simulink model "suspension7DOF"  (R2025b)
settings: Solver=ode5  StartTime=0.0  StopTime=10.0  FixedStep=0.001  RelTol=1e-3
InitFcn:
  | % 悬架参数
  | ksfl =  20000;
  | ksfr = ksfl;
  | ksrl =  20000;
  | ksrr = ksrl;
  | 
  | csfl = 1100;
  | csfr = 1100;
  | csrl = 1100;
  | csrr = 1100;
undefined symbols (not defined in the file): road
settings Model: Creator=23649  LastModifiedBy=23649

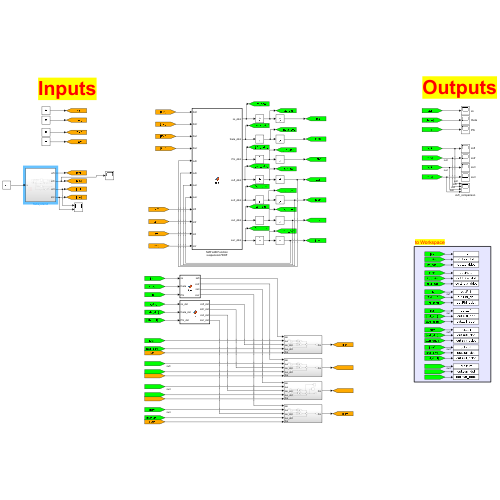
[thumbnail: Simulink's stored preview of the top-level diagram]
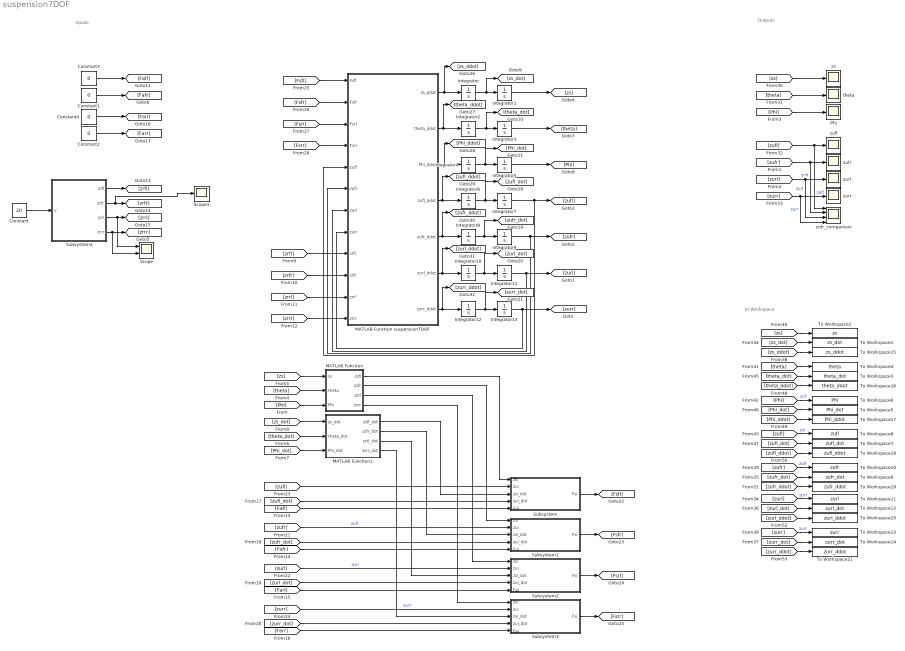
== system suspension7DOF ==
  note: Inputs
  note: Outputs
  note: to Workspace
  Constant : Constant  Value=20
  Constant{1..4} (4 alike) : Constant  Value=0
  Integrator{,1..13} (14 alike) : Integrator
  MATLAB Function : MATLAB Function  TreatAsAtomicUnit=on
  MATLAB Function suspension7DOF : MATLAB Function  TreatAsAtomicUnit=on
  MATLAB Function1 : MATLAB Function  TreatAsAtomicUnit=on
  Phi : Scope
      settings: ActiveDisplayYMinimum=-0.0087264176221422858  ActiveDisplayYMaximum=0.021115769306995449  DataLoggingVariableName=ScopeData7
  Scope : Scope  NumInputPorts=2
      settings: ActiveDisplayYMinimum=-0.0707302288699563  ActiveDisplayYMaximum=0.0028881749124079481  DataLoggingVariableName=ScopeData10
  Scope1 : Scope
      settings: ActiveDisplayYMinimum=-1  ActiveDisplayYMaximum=1  DataLoggingVariableName=ScopeData11
  Subsystem : Subsystem
  Subsystem1 : Subsystem
  Subsystem2 : Subsystem
  Subsystem3 : Subsystem
  Subsystem4 : Subsystem
  To Workspace1 : ToWorkspace  VariableName=zs_dot  SampleTime=-1
  To Workspace10 : ToWorkspace  VariableName=zufr  SampleTime=-1
  To Workspace11 : ToWorkspace  VariableName=zurl  SampleTime=-1
  To Workspace12 : ToWorkspace  VariableName=zurl_dot  SampleTime=-1
  To Workspace13 : ToWorkspace  VariableName=zurr  SampleTime=-1
  To Workspace14 : ToWorkspace  VariableName=zurr_dot  SampleTime=-1
  To Workspace15 : ToWorkspace  VariableName=zs_ddot  SampleTime=-1
  To Workspace16 : ToWorkspace  VariableName=theta_ddot  SampleTime=-1
  To Workspace17 : ToWorkspace  VariableName=Phi_ddot  SampleTime=-1
  To Workspace18 : ToWorkspace  VariableName=zufl_ddot  SampleTime=-1
  To Workspace19 : ToWorkspace  VariableName=zufr_ddot  SampleTime=-1
  To Workspace2 : ToWorkspace  VariableName=zs  SampleTime=-1
  To Workspace20 : ToWorkspace  VariableName=zurl_ddot  SampleTime=-1
  To Workspace21 : ToWorkspace  VariableName=zurr_ddot  SampleTime=-1
  To Workspace3 : ToWorkspace  VariableName=theta_dot  SampleTime=-1
  To Workspace4 : ToWorkspace  VariableName=theta  SampleTime=-1
  To Workspace5 : ToWorkspace  VariableName=Phi_dot  SampleTime=-1
  To Workspace6 : ToWorkspace  VariableName=Phi  SampleTime=-1
  To Workspace7 : ToWorkspace  VariableName=zufl_dot  SampleTime=-1
  To Workspace8 : ToWorkspace  VariableName=zufl  SampleTime=-1
  To Workspace9 : ToWorkspace  VariableName=zufr_dot  SampleTime=-1
  theta : Scope
      settings: ActiveDisplayYMinimum=-0.012479397367141442  ActiveDisplayYMaximum=0.012968504515283082
  zs : Scope
      settings: ActiveDisplayYMinimum=-0.038035702406532847  ActiveDisplayYMaximum=0.14136596040152494  DataLoggingVariableName=ScopeData2
  zufl : Scope
      settings: ActiveDisplayYMinimum=-1.3673893789653644  ActiveDisplayYMaximum=1.3691796129847056
  zufr : Scope
      settings: ActiveDisplayYMinimum=-1.3540132201466146  ActiveDisplayYMaximum=1.3380491130807826  DataLoggingVariableName=ScopeData5
  zufr_comparison : Scope  NumInputPorts=4
      settings: ActiveDisplayYMinimum=-0.078530307125556281  ActiveDisplayYMaximum=0.21658201066899388  DataLoggingVariableName=ScopeData4
  zurl : Scope
      settings: ActiveDisplayYMinimum=-1.3540132201466146  ActiveDisplayYMaximum=1.3380491130807826  DataLoggingVariableName=ScopeData6
  zurr : Scope
      settings: ActiveDisplayYMinimum=-1.3540132201466146  ActiveDisplayYMaximum=1.3380491130807826  DataLoggingVariableName=ScopeData3
  wires:
  Constant3/1 -> [Fafl]
  Constant1/1 -> [Fafr]
  [zs] -> zs/1
  [theta] -> theta/1
  [zufl] -> zufl/1, zufr_comparison/1  "zufl"
  [zurr] -> zufr_comparison/4, zurr/1  "zurr"
  MATLAB Function suspension7DOF/7(zurr_ddot) -> Integrator12/1, [zurr_ddot]
  MATLAB Function suspension7DOF/6(zurl_ddot) -> Integrator10/1, [zurl_ddot]
  MATLAB Function suspension7DOF/5(zufr_ddot) -> [zufr_ddot], Integrator8/1
  MATLAB Function suspension7DOF/4(zufl_ddot) -> Integrator6/1, [zufl_ddot]
  MATLAB Function suspension7DOF/1(zs_ddot) -> [zs_ddot], Integrator/1
  Integrator/1 -> [zs_dot], Integrator1/1
  Integrator2/1 -> [theta_dot], Integrator3/1
  Integrator4/1 -> [Phi_dot], Integrator5/1
  Integrator6/1 -> Integrator7/1, [zufl_dot]
  Integrator8/1 -> [zufr_dot], Integrator9/1
  Integrator10/1 -> [zurl_dot], Integrator11/1
  Integrator12/1 -> [zurr_dot], Integrator13/1
  MATLAB Function suspension7DOF/3(Phi_ddot) -> [Phi_ddot], Integrator4/1
  MATLAB Function suspension7DOF/2(theta_ddot) -> Integrator2/1, [theta_ddot]
  Integrator13/1 -> [zurr], MATLAB Function suspension7DOF/8(zurr)
  Integrator11/1 -> [zurl], MATLAB Function suspension7DOF/7(zurl)
  Integrator9/1 -> [zufr], MATLAB Function suspension7DOF/6(zufr)
  Integrator7/1 -> [zufl], MATLAB Function suspension7DOF/5(zufl)
  [zufr] -> zufr_comparison/2, zufr/1  "zufr"
  [zurl] -> zurl/1, zufr_comparison/3  "zurl"
  [Phi] -> Phi/1
  Integrator5/1 -> [Phi]
  Integrator3/1 -> [theta]
  Integrator1/1 -> [zs]
  [zs] -> MATLAB Function/1(zs)
  [theta] -> MATLAB Function/2(theta)
  [Phi] -> MATLAB Function/3(Phi)
  [zs_dot] -> MATLAB Function1/1(zs_dot)
  [theta_dot] -> MATLAB Function1/2(theta_dot)
  [Phi_dot] -> MATLAB Function1/3(Phi_dot)
  [zrfl] -> MATLAB Function suspension7DOF/9(zrfl)
  [zrfr] -> MATLAB Function suspension7DOF/10(zrfr)
  [zrrl] -> MATLAB Function suspension7DOF/11(zrrl)
  [zrrr] -> MATLAB Function suspension7DOF/12(zrrr)
  MATLAB Function/1(zsfl) -> Subsystem/1(zsi)
  [zufl] -> Subsystem/2(zui)
  [zufl_dot] -> Subsystem/4(zui_dot)
  [Fafl] -> Subsystem/5(Fai)
  Subsystem/1(Fsi) -> [Fsfl]
  Constant2/1 -> [Farr]
  Constant4/1 -> [Farl]
  MATLAB Function/2(zsfr) -> Subsystem1/1(zsi)
  MATLAB Function/3(zsrl) -> Subsystem2/1(zsi)
  MATLAB Function/4(zsrr) -> Subsystem3/1(zsi)
  MATLAB Function1/1(zsfl_dot) -> Subsystem/3(zsi_dot)
  MATLAB Function1/2(zsfr_dot) -> Subsystem1/3(zsi_dot)
  MATLAB Function1/3(zsrl_dot) -> Subsystem2/3(zsi_dot)
  MATLAB Function1/4(zsrr_dot) -> Subsystem3/3(zsi_dot)
  [zufr_dot] -> Subsystem1/4(zui_dot)
  [zurr_dot] -> Subsystem3/4(zui_dot)
  [zurl_dot] -> Subsystem2/4(zui_dot)
  [Farr] -> Subsystem3/5(Fai)
  [Farl] -> Subsystem2/5(Fai)
  [Fafr] -> Subsystem1/5(Fai)
  [zufr] -> Subsystem1/2(zui)  "zufr"
  [zurl] -> Subsystem2/2(zui)  "zurl"
  [zurr] -> Subsystem3/2(zui)  "zurr"
  Subsystem3/1(Fsi) -> [Fsrr]
  Subsystem2/1(Fsi) -> [Fsrl]
  Subsystem1/1(Fsi) -> [Fsfr]
  [Fsfl] -> MATLAB Function suspension7DOF/1(Fsfl)
  [Fsfr] -> MATLAB Function suspension7DOF/2(Fsfr)
  [Fsrl] -> MATLAB Function suspension7DOF/3(Fsrl)
  [Fsrr] -> MATLAB Function suspension7DOF/4(Fsrr)
  Subsystem4/1(zrfl) -> [zrfl]
  Subsystem4/2(zrfr) -> Scope1/1, [zrfr]
  Subsystem4/3(zrrl) -> Scope/1, [zrrl]
  Constant/1 -> Subsystem4/1(v)
  [zufl] -> To Workspace8/1  "zur"
  [zs] -> To Workspace2/1
  [zufl_dot] -> To Workspace7/1
  [Phi] -> To Workspace6/1  "zuf"
  [theta] -> To Workspace4/1
  [Phi_dot] -> To Workspace5/1
  [theta_dot] -> To Workspace3/1
  [zs_dot] -> To Workspace1/1
  [zurr_dot] -> To Workspace14/1
  [zurr] -> To Workspace13/1  "zurr"
  [zurl_dot] -> To Workspace12/1
  [zurl] -> To Workspace11/1  "zurl"
  [zufr_dot] -> To Workspace9/1
  [zufr] -> To Workspace10/1  "zufr"
  [zs_ddot] -> To Workspace15/1
  [theta_ddot] -> To Workspace16/1
  [Phi_ddot] -> To Workspace17/1
  [zufl_ddot] -> To Workspace18/1
  [zufr_ddot] -> To Workspace19/1
  [zurl_ddot] -> To Workspace20/1
  [zurr_ddot] -> To Workspace21/1
  Subsystem4/4(zrrr) -> Scope/2, [zrrr]

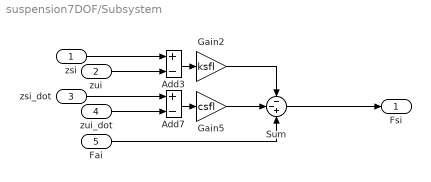
== system suspension7DOF/Subsystem ==
  zsi : Inport
  zui : Inport  Port=2
  zsi_dot : Inport  Port=3
  zui_dot : Inport  Port=4
  Fai : Inport  Port=5
  Add3 : Sum  Inputs=+-
  Add7 : Sum  Inputs=+-
  Gain2 : Gain  Gain=ksfl
  Gain5 : Gain  Gain=csfl
  Sum : Sum  Inputs=--+
  Fsi : Outport
  wires:
  Gain2/1 -> Sum/1
  zsi_dot/1 -> Add7/1
  zsi/1 -> Add3/1
  Add7/1 -> Gain5/1
  zui/1 -> Add3/2
  Add3/1 -> Gain2/1
  Gain5/1 -> Sum/2
  Fai/1 -> Sum/3
  Sum/1 -> Fsi/1
  zui_dot/1 -> Add7/2

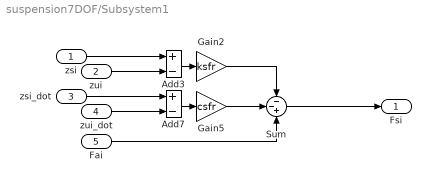
== system suspension7DOF/Subsystem1 ==
  zsi : Inport
  zui : Inport  Port=2
  zsi_dot : Inport  Port=3
  zui_dot : Inport  Port=4
  Fai : Inport  Port=5
  Add3 : Sum  Inputs=+-
  Add7 : Sum  Inputs=+-
  Gain2 : Gain  Gain=ksfr
  Gain5 : Gain  Gain=csfr
  Sum : Sum  Inputs=--+
  Fsi : Outport
  wires:
  zui_dot/1 -> Add7/2
  Sum/1 -> Fsi/1
  Fai/1 -> Sum/3
  Gain5/1 -> Sum/2
  Add3/1 -> Gain2/1
  zui/1 -> Add3/2
  Add7/1 -> Gain5/1
  zsi/1 -> Add3/1
  zsi_dot/1 -> Add7/1
  Gain2/1 -> Sum/1

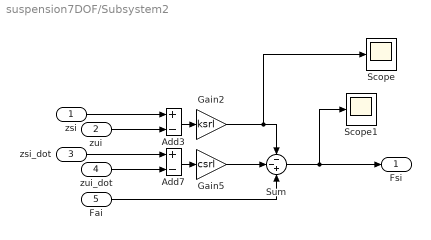
== system suspension7DOF/Subsystem2 ==
  zsi : Inport
  zui : Inport  Port=2
  zsi_dot : Inport  Port=3
  zui_dot : Inport  Port=4
  Fai : Inport  Port=5
  Add3 : Sum  Inputs=+-
  Add7 : Sum  Inputs=+-
  Gain2 : Gain  Gain=ksrl
  Gain5 : Gain  Gain=csrl
  Scope : Scope
      settings: ActiveDisplayYMinimum=-1  ActiveDisplayYMaximum=1  DataLoggingVariableName=ScopeData8
  Scope1 : Scope
      settings: ActiveDisplayYMinimum=-8980.6897654374643  ActiveDisplayYMaximum=18965.2502378485  DataLoggingVariableName=ScopeData9
  Sum : Sum  Inputs=--+
  Fsi : Outport
  wires:
  Gain2/1 -> Scope/1, Sum/1
  zsi_dot/1 -> Add7/1
  zsi/1 -> Add3/1
  Add7/1 -> Gain5/1
  zui/1 -> Add3/2
  Add3/1 -> Gain2/1
  Gain5/1 -> Sum/2
  Fai/1 -> Sum/3
  Sum/1 -> Scope1/1, Fsi/1
  zui_dot/1 -> Add7/2

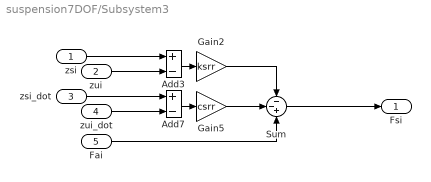
== system suspension7DOF/Subsystem3 ==
  zsi : Inport
  zui : Inport  Port=2
  zsi_dot : Inport  Port=3
  zui_dot : Inport  Port=4
  Fai : Inport  Port=5
  Add3 : Sum  Inputs=+-
  Add7 : Sum  Inputs=+-
  Gain2 : Gain  Gain=ksrr
  Gain5 : Gain  Gain=csrr
  Sum : Sum  Inputs=--+
  Fsi : Outport
  wires:
  zui_dot/1 -> Add7/2
  Sum/1 -> Fsi/1
  Fai/1 -> Sum/3
  Gain5/1 -> Sum/2
  Add3/1 -> Gain2/1
  zui/1 -> Add3/2
  Add7/1 -> Gain5/1
  zsi/1 -> Add3/1
  zsi_dot/1 -> Add7/1
  Gain2/1 -> Sum/1

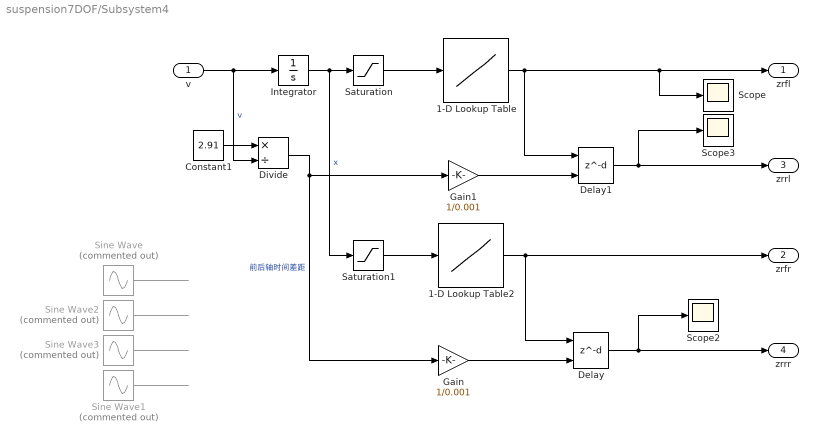
== system suspension7DOF/Subsystem4 ==
  v : Inport
  1-D Lookup Table : Lookup_n-D  NumberOfTableDimensions=1  BreakpointsForDimension1=road.x  Table=road.z_L  ExtrapMethod=Clip  InternalRulePriority=Speed  RndMeth=Simplest
  1-D Lookup Table2 : Lookup_n-D  NumberOfTableDimensions=1  BreakpointsForDimension1=road.x  Table=road.z_R  ExtrapMethod=Clip  InternalRulePriority=Speed  RndMeth=Simplest
  Constant1 : Constant  Value=2.91
  Delay : Delay  DelayLengthSource=Input port  DelayLength=1  DelayLengthUpperLimit=1000  InputProcessing=Columns as channels (frame based)
      settings: InputPortMap=u0,p1
  Delay1 : Delay  DelayLengthSource=Input port  DelayLength=1  DelayLengthUpperLimit=1000  InputProcessing=Columns as channels (frame based)
      settings: InputPortMap=u0,p1
  Divide : Product  Inputs=*/
  Gain : Gain  Gain=1/0.001
  Gain1 : Gain  Gain=1/0.001
  Integrator : Integrator
  Saturation : Saturate  UpperLimit=road.L-road.dx  LowerLimit=0
  Saturation1 : Saturate  UpperLimit=road.L-road.dx  LowerLimit=0
  Scope : Scope
      settings: ActiveDisplayYMinimum=-1  ActiveDisplayYMaximum=1  DataLoggingVariableName=ScopeData12
  Scope2 : Scope
      settings: ActiveDisplayYMinimum=-1  ActiveDisplayYMaximum=1  DataLoggingVariableName=ScopeData14
  Scope3 : Scope
      settings: ActiveDisplayYMinimum=-0.089220015836879121  ActiveDisplayYMaximum=0.19824348779036427  DataLoggingVariableName=ScopeData15
  Sine Wave : Sin  Commented=on  Frequency=5  SampleTime=0
  Sine Wave1 : Sin  Commented=on  Frequency=5  Phase=7  SampleTime=0
  Sine Wave2 : Sin  Commented=on  Frequency=5  SampleTime=0
  Sine Wave3 : Sin  Commented=on  Frequency=5  Phase=12  SampleTime=0
  zrfl : Outport
  zrfr : Outport  Port=2
  zrrl : Outport  Port=3
  zrrr : Outport  Port=4
  wires:
  v/1 -> Integrator/1, Divide/2  "v"
  Integrator/1 -> Saturation/1, Saturation1/1  "x"
  Saturation/1 -> 1-D Lookup Table/1
  Saturation1/1 -> 1-D Lookup Table2/1
  Sine Wave2/1 -> ?
  Sine Wave1/1 -> ?
  Sine Wave/1 -> ?
  Sine Wave3/1 -> ?
  Delay/1 -> Scope2/1, zrrr/1
  Constant1/1 -> Divide/1
  Divide/1 -> Gain1/1, Gain/1  "前后轴时间差距"
  Gain/1 -> Delay/2
  1-D Lookup Table2/1 -> Delay/1, zrfr/1
  1-D Lookup Table/1 -> Delay1/1, Scope/1, zrfl/1
  Gain1/1 -> Delay1/2
  Delay1/1 -> zrrl/1, Scope3/1

== matlab function suspension7DOF/MATLAB Function ==
  data: zs input; zsfl output; theta input; Phi input; zsfr output; zsrl output; zsrr output
function [zsfl, zsfr, zsrl, zsrr] = fcn(zs, theta, Phi)
    
    lf = 1110*0.001;
    L = 2866*0.001;
    % lr = L-lf;
    lr = lf;
    Bf = 1550*0.001;
    Br = Bf;


    zsfl = zs - lf*theta + Bf/2*Phi;
    zsfr = zs - lf*theta - Bf/2*Phi;
    zsrl = zs + lr*theta + Br/2*Phi;
    zsrr = zs + lr*theta - Br/2*Phi;

end

== matlab function suspension7DOF/MATLAB Function suspension7DOF ==
  data: Fsfl input; zs_ddot output; theta_ddot output; Phi_ddot output; zufl_ddot output; zufr_ddot output; zurl_ddot output; zurr_ddot output; Fsfr input; Fsrl input; Fsrr input; zufl input; zufr input; zurl input; zurr input; zrfl input; zrfr input; zrrl input; zrrr input
function [zs_ddot,theta_ddot,Phi_ddot,zufl_ddot,zufr_ddot,zurl_ddot,zurr_ddot] = fcn(Fsfl,Fsfr,Fsrl,Fsrr,zufl,zufr,zurl,zurr,zrfl,zrfr,zrrl,zrrr)
    % 物理参数
    m_s = 1370;
    Iy = 1972.8;
    Ix = 671.3;
    lf = 1110*0.001;
    L = 2866*0.001;
    lr = L-lf;
    Bf = 1550*0.001;
    Br = Bf;
    m_ufl = 89.9/2;
    m_ufr = m_ufl;
    m_url = 65.2/2;
    m_urr = m_url;
    ktfl = 268000;
    ktfr = ktfl;
    ktrl = 208000;
    ktrr = ktrl;



    % 7DOF 悬架-整车动力学模型
    % 整车 垂向、俯仰、侧倾
    zs_ddot = (Fsfl+Fsfr+Fsrl+Fsrr) / m_s;
    theta_ddot = (-(Fsfl+Fsfr)*lf + (Fsrl+Fsrr)*lr) / Iy;
    Phi_ddot = ((Fsfl-Fsfr)*Bf + (Fsrl-Fsrr)*Br) / (2*Ix);
    
    % 四个车轮
    zufl_ddot = (-Fsfl - ktfl*(zufl-zrfl)) / m_ufl;
    zufr_ddot = (-Fsfr - ktfr*(zufr-zrfr)) / m_ufr;
    zurl_ddot = (-Fsrl - ktrl*(zurl-zrrl)) / m_url;
    zurr_ddot = (-Fsrr - ktrr*(zurr-zrrr)) / m_urr;

end

== matlab function suspension7DOF/MATLAB Function1 ==
  data: zs_dot input; zsfl_dot output; theta_dot input; Phi_dot input; zsfr_dot output; zsrl_dot output; zsrr_dot output
function [zsfl_dot, zsfr_dot, zsrl_dot, zsrr_dot] = fcn(zs_dot, theta_dot, Phi_dot)
    
    lf = 1110*0.001;
    L = 2866*0.001;
    lr = L-lf;
    Bf = 1550*0.001;
    Br = Bf;


    zsfl_dot = zs_dot - lf*theta_dot + Bf/2*Phi_dot;
    zsfr_dot = zs_dot - lf*theta_dot - Bf/2*Phi_dot;
    zsrl_dot = zs_dot + lr*theta_dot + Br/2*Phi_dot;
    zsrr_dot = zs_dot + lr*theta_dot - Br/2*Phi_dot;

end
